simulink model "Approach1"  (R2018b)
settings: Solver=VariableStepAuto  StartTime=0.0  StopTime=3.0  RelTol=1e-3
libraries: vrlib x1
settings Model: Creator=martinandersen  LastModifiedBy=martinandersen

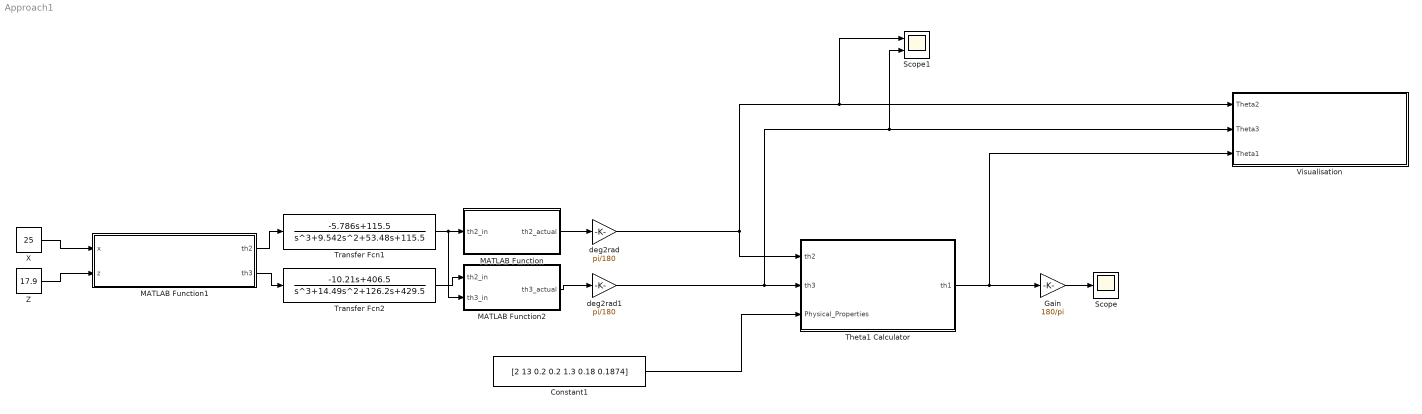
== system Approach1 ==
  Constant1 : Constant  Value=[2 13 0.2 0.2 1.3 0.18 0.1874]
  Gain : Gain  Gain=180/pi
  MATLAB Function : MATLAB Function  TreatAsAtomicUnit=on
  MATLAB Function1 : MATLAB Function  TreatAsAtomicUnit=on
  MATLAB Function2 : MATLAB Function  TreatAsAtomicUnit=on
  Scope : Scope
  Scope1 : Scope  NumInputPorts=2
  Theta1 Calculator : MATLAB Function  TreatAsAtomicUnit=on
  Transfer Fcn1 : TransferFcn  Numerator=[-5.786 115.5]  Denominator=[1 9.542 53.48 115.5]
  Transfer Fcn2 : TransferFcn  Numerator=[-10.21 406.5]  Denominator=[1 14.49 126.2 429.5]
  Visualisation : Subsystem
  X : Constant  Value=25
  Z : Constant  Value=17.9
  deg2rad : Gain  Gain=pi/180
  deg2rad1 : Gain  Gain=pi/180
  wires:
  Transfer Fcn2/1 -> MATLAB Function2/1(th2_in)
  Constant1/1 -> Theta1 Calculator/3(Physical_Properties)
  Transfer Fcn1/1 -> MATLAB Function/1(th2_in), MATLAB Function2/2(th3_in)
  MATLAB Function1/1(th2) -> Transfer Fcn1/1
  MATLAB Function1/2(th3) -> Transfer Fcn2/1
  X/1 -> MATLAB Function1/1(x)
  Z/1 -> MATLAB Function1/2(z)
  Theta1 Calculator/1(th1) -> Gain/1, Visualisation/3(Theta1)
  Gain/1 -> Scope/1
  deg2rad/1 -> Theta1 Calculator/1(th2), Visualisation/1(Theta2), Scope1/1
  deg2rad1/1 -> Visualisation/2(Theta3), Scope1/2, Theta1 Calculator/2(th3)
  MATLAB Function/1(th2_actual) -> deg2rad/1
  MATLAB Function2/1(th3_actual) -> deg2rad1/1

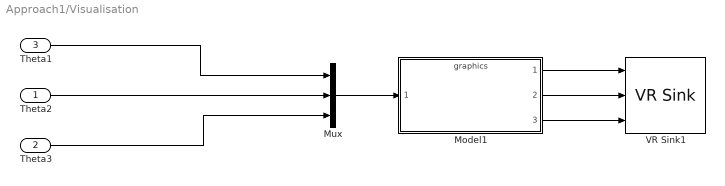
== system Approach1/Visualisation ==
  Theta2 : Inport
  Theta3 : Inport  Port=2
  Theta1 : Inport  Port=3
  Model1 : ModelReference  ModelNameDialog=graphics.slx  SimulationMode=Normal  ModelReferenceVersion=1.13
  Mux : Mux  Inputs=3
  VR Sink1 : vrlib/VR Sink  InstantiateOnLoad=on  SampleTime=0.1  ViewEnable=on  RemoteChange=off  RemoteView=off  FieldsWritten=JOINT_1.rotation.4.1.1.double#JOINT_2.rotation.4.1.1.double#JOINT_3.rotation.4.1.1.double  WorldFileName=Pendel3D0.wrl  AutoView=off  VideoDimensions=[]  AllowVariableSize=off  FigureProperties="{'Position', 'Name', 'Viewpoint', 'CameraBound', 'CameraDirection', 'CameraPosition', 'CameraUpVector', 'ZoomFactor', 'Antialiasing', 'Headlight', 'Lighting', 'NavPanel', 'Sound', 'StatusBar', 'Stereo3D', 'Stereo3DCameraOffset', 'Stereo3DHIT', 'ToolBar', 'Textures', 'Transparency', 'Triad', 'Wireframe', 'NavZones', 'NavMode', 'NavSpeed', 'CaptureFileFormat', 'CaptureFileName', 'Record2DCompressMethod', 'Record2DCompressQuality', 'Record2D', 'Record2DFileName', 'Record2DFPS'; [5.0000000000000000e+00   9.5000000000000000e+01   5.7600000000000000e+02   3.5000000000000000e+02], '', '', 'on', [0.0000000000000000e+00   0.0000000000000000e+00  -1.0000000000000000e+00], [0.0000000000000000e+00   0.0000000000000000e+00   1.0000000000000000e+01], [0.0000000000000000e+00   1.0000000000000000e+00   0.0000000000000000e+00], [1.0000000000000000e+00], 'on', 'on', 'on', 'halfbar', 'on', 'on', 'off', [1.0000000149011612e-01], [0.0000000000000000e+00], 'on', 'on', 'on', 'none', 'off', 'off', 'fly', 'normal', 'tif', '%f_anim_%n.tif', 'auto', [7.5000000000000000e+01], 'off', '%f_anim_%n.avi', 'auto'}"
      settings: SourceProductBaseCode=VR
  wires:
  Model1/1 -> VR Sink1/1
  Model1/2 -> VR Sink1/2
  Theta3/1 -> Mux/3
  Theta2/1 -> Mux/2
  Model1/3 -> VR Sink1/3
  Theta1/1 -> Mux/1
  Mux/1 -> Model1/1

== matlab function Approach1/MATLAB Function1 ==
  data: x input; th2 output; z input; th3 output
function [th2,th3] = InverseGeometrical(x,z)

L1 = 18.2;
L2 = 18.74; % calculated and verified by measurement. From one rotating joint to the other.


D = (L1^2 + L2^2 - (x^2 + z^2))/(2*L1*L2);
th3 = 180 - atan2d(-sqrt(1-D^2),D);

alpha = atan2d(L2*sind(th3),L1 + L2*cosd(th3));

beta = atan2d(z,x);
th2 = beta - alpha;

th2 = 90 - th2;
th3 = 360 - th3;
end

== matlab function Approach1/Theta1 Calculator ==
  data: th2 input; th1 output; th3 input; Physical_Properties input
function th1 = fcn(th2, th3, Physical_Properties)

m1      = Physical_Properties(2);
m2      = Physical_Properties(3);
m3      = Physical_Properties(4);

l1      = Physical_Properties(5);
l2      = Physical_Properties(6);
l3      = Physical_Properties(7);

mt = m1 + m2 + m3;

th1 = real(-log(((l3*m3 + l2*m2*exp(th3*1i) + 2*l2*m3*exp(th3*1i) + l1*m1*exp(th2*1i)*exp(th3*1i) + 2*l1*m2*exp(th2*1i)*exp(th3*1i) + 2*l1*m3*exp(th2*1i)*exp(th3*1i))*(l1*m1 + 2*l1*m2 + 2*l1*m3 + l2*m2*exp(th2*1i) + 2*l2*m3*exp(th2*1i) + l3*m3*exp(th2*1i)*exp(th3*1i)))^(1/2)/(l1*m1*exp((th2*1i)/2)*exp((th3*1i)/2) + 2*l1*m2*exp((th2*1i)/2)*exp((th3*1i)/2) + 2*l1*m3*exp((th2*1i)/2)*exp((th3*1i)/2) + l2*m2*exp((th3*1i)/2)*exp((th2*3i)/2) + 2*l2*m3*exp((th3*1i)/2)*exp((th2*3i)/2) + l3*m3*exp((th2*3i)/2)*exp((th3*3i)/2)))*1i);

== matlab function Approach1/MATLAB Function ==
  data: th2_in input; th2_actual output
function th2_actual = fcn(th2_in)

joint2offset = 32.94-90;

th2_actual = (th2_in-joint2offset)*-1;

== matlab function Approach1/MATLAB Function2 ==
  data: th2_in input; th3_actual output; th3_in input
function th3_actual = fcn(th2_in, th3_in)

joint2offset = 32.94-90;
joint3offset = 180-46.1;

th3_actual = (th3_in-joint3offset)+(th2_in-joint2offset)
